simulink model "radar_simulation"  (R2022a)
settings: Solver=VariableStepAuto  StartTime=0.0  StopTime=500000  RelTol=1e-3
model workspace (MAT data in the model file):
  Center_Frequency = Simulink.Parameter
  Center_Frequency.Value = 62000000000
  Center_Frequency.DataType = 'auto'
  Center_Frequency.Min = 60000000000
  Center_Frequency.Max = 64000000000
  Center_Frequency.DocUnits = 'Hz'
  Center_Frequency.Complexity = 'real'
  Center_Frequency.Dimensions = [1 1]
  Chirps_Per_Sequence = Simulink.Parameter
  Chirps_Per_Sequence.Value = 128
  Chirps_Per_Sequence.DataType = 'auto'
  Chirps_Per_Sequence.Min = 1
  Chirps_Per_Sequence.Complexity = 'real'
  Chirps_Per_Sequence.Dimensions = [1 1]
  Close_Rate = Simulink.Parameter
  Close_Rate.Value = 10
  Close_Rate.DataType = 'auto'
  Close_Rate.DocUnits = 'm/s'
  Close_Rate.Complexity = 'real'
  Close_Rate.Dimensions = [1 1]
  Initial_Range = Simulink.Parameter
  Initial_Range.Value = 15
  Initial_Range.DataType = 'auto'
  Initial_Range.DocUnits = 'm'
  Initial_Range.Complexity = 'real'
  Initial_Range.Dimensions = [1 1]
  Max_Range = Simulink.Parameter
  Max_Range.Value = 100
  Max_Range.DataType = 'auto'
  Max_Range.Min = 0
  Max_Range.DocUnits = 'm'
  Max_Range.Complexity = 'real'
  Max_Range.Dimensions = [1 1]
  Range_Resolution = Simulink.Parameter
  Range_Resolution.Value = 1
  Range_Resolution.DataType = 'auto'
  Range_Resolution.Min = 0
  Range_Resolution.DocUnits = 'm'
  Range_Resolution.Complexity = 'real'
  Range_Resolution.Dimensions = [1 1]
  Samples_Per_Chirp = Simulink.Parameter
  Samples_Per_Chirp.Value = 1024
  Samples_Per_Chirp.DataType = 'auto'
  Samples_Per_Chirp.Min = 1
  Samples_Per_Chirp.Complexity = 'real'
  Samples_Per_Chirp.Dimensions = [1 1]
undefined symbols (not defined in the file or in its folder): aperture2gain, freq2wavelen, physconst
libraries: phasedenvlib x4, phaseddetectlib x2, phasedtxrxlib x2, phasedwavlib x1
settings Model: SimulationMode=accelerator  Creator=mhatch  LastModifiedBy=mhatch

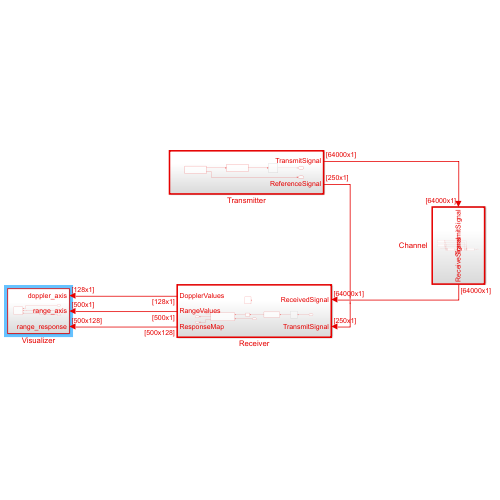
[thumbnail: Simulink's stored preview of the top-level diagram]
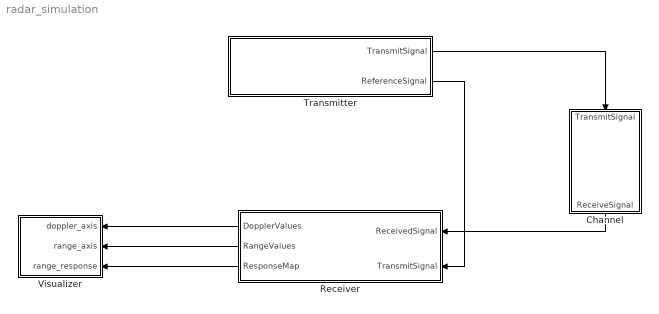
== system radar_simulation ==
  Channel : Subsystem  TreatAsAtomicUnit=on
  Receiver : Subsystem  TreatAsAtomicUnit=on
  Transmitter : Subsystem  TreatAsAtomicUnit=on
  Visualizer : Subsystem
  wires:
  Transmitter/1(TransmitSignal) -> Channel/1(TransmitSignal)
  Channel/1(ReceiveSignal) -> Receiver/1(ReceivedSignal)
  Receiver/1(DopplerValues) -> Visualizer/1(doppler_axis)
  Receiver/2(RangeValues) -> Visualizer/2(range_axis)
  Receiver/3(ResponseMap) -> Visualizer/3(range_response)
  Transmitter/2(ReferenceSignal) -> Receiver/2(TransmitSignal)

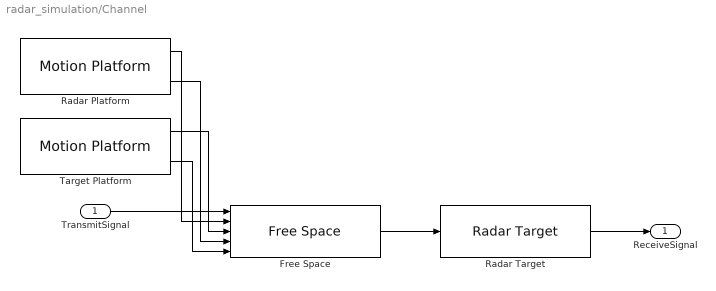
== system radar_simulation/Channel ==
  TransmitSignal : Inport
  Free Space : phasedenvlib/Free Space  PropagationSpeed=physconst( 'LightSpeed' )  OperatingFrequency=60e9  TwoWayPropagation=on  SampleRateFromInputCheckbox=on  SampleRate=1e6  MaximumDistanceSource=Property  MaximumDistance=100  MaximumNumInputSamplesSource=Auto  MaximumNumInputSamples=1000  SimulateUsing=Code generation
      settings: SourceProductBaseCode=AR
  Radar Platform : phasedenvlib/Motion Platform  MotionModel=Velocity  InitialPosition=[ 0; 0; 0.5 ]  InitialVelocity=[ 0; 0; 0 ]  VelocitySource=Property  Velocity=[0; 0; 0]  AccelerationSource=Property  Acceleration=[0;0;0]  CustomTrajectory=[ 0, 0, 0, 0, 0, 0, 0; 1, 0, 0, 0, 0, 0, 0 ]  ScanMode=None  InitialScanAngle=0  AzimuthSpan=[ -60, 60 ]  AzimuthScanRate=10  InitialOrientationAxes=eye( 3 )  OrientationAxesOutputPort=off  ElapsedTimeSource=Auto  SampleRateFromInputCheckbox=on  SampleRate=1e6  SimulateUsing=Code generation
      settings: SourceProductBaseCode=AR
  Radar Target : phasedenvlib/Radar Target  EnablePolarization=off  Mode=Monostatic  MeanRCSSource=Property  ScatteringMatrixSource=Property  MeanRCS=min(pow2db(20), 0.1)  ScatteringMatrix=eye( 2 )  Model=Nonfluctuating  PropagationSpeed=physconst( 'LightSpeed' )  OperatingFrequency=60e9  SeedSource=Auto  Seed=0  SimulateUsing=Code generation
      settings: SourceProductBaseCode=AR
  Target Platform : phasedenvlib/Motion Platform  MotionModel=Velocity  InitialPosition=[ 20; 0; 0.5 ]  InitialVelocity=[ 0; 0; 0 ]  VelocitySource=Property  Velocity=[5; 0; 0]  AccelerationSource=Property  Acceleration=[0;0;0]  CustomTrajectory=[ 0, 0, 0, 0, 0, 0, 0; 1, 0, 0, 0, 0, 0, 0 ]  ScanMode=None  InitialScanAngle=0  AzimuthSpan=[ -60, 60 ]  AzimuthScanRate=10  InitialOrientationAxes=eye( 3 )  OrientationAxesOutputPort=off  ElapsedTimeSource=Auto  SampleRateFromInputCheckbox=on  SampleRate=1e6  SimulateUsing=Code generation
      settings: SourceProductBaseCode=AR
  ReceiveSignal : Outport
  wires:
  Radar Platform/1 -> Free Space/2
  Radar Platform/2 -> Free Space/4
  Target Platform/2 -> Free Space/5
  Target Platform/1 -> Free Space/3
  TransmitSignal/1 -> Free Space/1
  Free Space/1 -> Radar Target/1
  Radar Target/1 -> ReceiveSignal/1

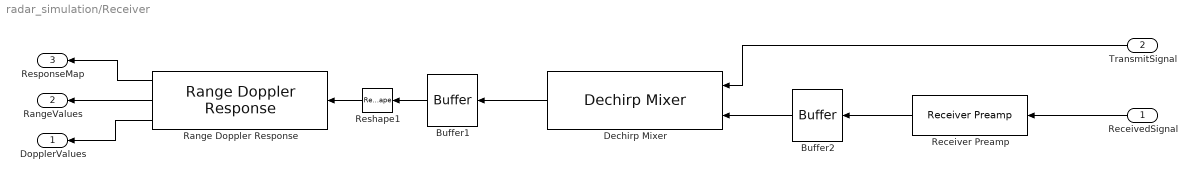
== system radar_simulation/Receiver ==
  ReceivedSignal : Inport
  TransmitSignal : Inport  Port=2
  Buffer1 : Buffer  N=92160  OutputFrames=off
  Buffer2 : Buffer  N=720  OutputFrames=off
  Dechirp Mixer : phaseddetectlib/Dechirp Mixer
      settings: SourceProductBaseCode=AR
  Range Doppler Response : phaseddetectlib/Range Doppler Response  RangeMethod=FFT  PropagationSpeed=physconst( 'lightspeed' )  SampleRateFromInputCheckbox=off  SampleRate=15e6  SweepSlope=135e6 / 45e-6  DechirpInput=off  RangeFFTLengthSource=Property  RangeFFTLength=2048  RangeWindow=None  RangeSidelobeAttenuation=30  CustomRangeWindow=@hamming  ReferenceRangeCentered=on  ReferenceRange=0  MaximumNumInputSamplesSource=Auto  MaximumNumInputSamples=100  PRFSource=Auto  PRF=10e3  DopplerFFTLengthSource=Property  DopplerFFTLength=256  DopplerWindow=None  DopplerSidelobeAttenuation=30  CustomDopplerWindow=@hamming  DopplerOutput=Speed  OperatingFrequency=60e9  SimulateUsing=Code generation
      settings: SourceProductBaseCode=AR
  Receiver Preamp : phasedtxrxlib/Receiver Preamp  Gain="15 +  + aperture2gain(.0045^2, freq2wavelen(60e9, 300e6))"  LossFactor=0  NoiseMethod=Noise temperature  NoiseFigure=4.5  ReferenceTemperature=290  SampleRateFromInputCheckbox=on  SampleRate=1e6  NoisePower=0  EnableInputPort=off  PhaseNoiseInputPort=off  SeedSource=Auto  Seed=0  SimulateUsing=Code generation
      settings: SourceProductBaseCode=AR
  Reshape1 : Reshape  OutputDimensionality=Customize  OutputDimensions=[(92160/128) 128]
  DopplerValues : Outport
  RangeValues : Outport  Port=2
  ResponseMap : Outport  Port=3
  wires:
  Range Doppler Response/1 -> ResponseMap/1
  Range Doppler Response/2 -> RangeValues/1
  Range Doppler Response/3 -> DopplerValues/1
  Reshape1/1 -> Range Doppler Response/1
  ReceivedSignal/1 -> Receiver Preamp/1
  Receiver Preamp/1 -> Buffer2/1
  Buffer2/1 -> Dechirp Mixer/2
  TransmitSignal/1 -> Dechirp Mixer/1
  Dechirp Mixer/1 -> Buffer1/1
  Buffer1/1 -> Reshape1/1

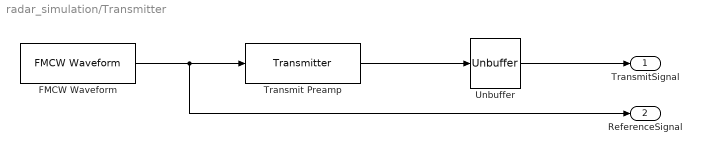
== system radar_simulation/Transmitter ==
  FMCW Waveform : phasedwavlib/FMCW Waveform  SampleRate=16e6  SweepTime=45e-6  SweepBandwidth=135e6  SweepDirection=Up  SweepInterval=Positive  OutputFormat=Sweeps  NumSamples=100  NumSweeps=1  SimulateUsing=Code generation
      settings: SourceProductBaseCode=AR
  Transmit Preamp : phasedtxrxlib/Transmitter  PeakPower=db2pow(10)  Gain=9 + aperture2gain(.0045^2, freq2wavelen(60e9, 300e6))  LossFactor=0  InUseOutputPort=off  CoherentOnTransmit=on  PhaseNoiseOutputPort=off  SeedSource=Auto  Seed=0  SimulateUsing=Code generation
      settings: SourceProductBaseCode=AR
  Unbuffer : Unbuffer
  TransmitSignal : Outport
  ReferenceSignal : Outport  Port=2
  wires:
  Transmit Preamp/1 -> Unbuffer/1
  Unbuffer/1 -> TransmitSignal/1
  FMCW Waveform/1 -> ReferenceSignal/1, Transmit Preamp/1

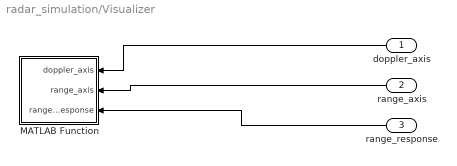
== system radar_simulation/Visualizer ==
  doppler_axis : Inport
  range_axis : Inport  Port=2
  range_response : Inport  Port=3
  MATLAB Function : MATLAB Function  TreatAsAtomicUnit=on
  wires:
  doppler_axis/1 -> MATLAB Function/1(doppler_axis)
  range_axis/1 -> MATLAB Function/2(range_axis)
  range_response/1 -> MATLAB Function/3(range_response)

== matlab function radar_simulation/Visualizer/MATLAB Function ==
  data: doppler_axis input; range_axis input; range_response input
function fcn(doppler_axis, range_axis, range_response)

coder.extrinsic('imagesc');

imagesc(doppler_axis, range_axis, mag2db(abs(range_response)));
xlabel('Speed (m/s)');
ylabel('Range (m)');
title('Range-Doppler Map');

end
